simulink model "CryoDet"  (R2015b)
settings: Solver=ode45  SolverMode=SingleTasking  StartTime=0.0  StopTime=1e-4  MaxStep=1e-9  RelTol=1e-3
values from neighbouring files (symbols this model uses):
  Fclk = Fadc    (= 307200000)    [setupCryoFPGAxray.m]
  freqBusAddrBits = 4    [setupCryoFPGAxray.m]
  noise = exp(2i*pi*rand(1, noiseLen))    [setupCryoFPGAxray.m]
  noiseLen = 128    [setupCryoFPGAxray.m]
  noiseSteps = 32    [setupCryoFPGAxray.m]
  Tclk = 1/Fclk    (= 3.25520833333e-09)    [setupCryoFPGAxray.m]
undefined symbols (not defined in the file or in its folder): AXI4, Lite, notch, notch2, notch3, notch4, xlipgetpartsetting
libraries: xbsIndex_r4 x1227
(part 2 of 9)

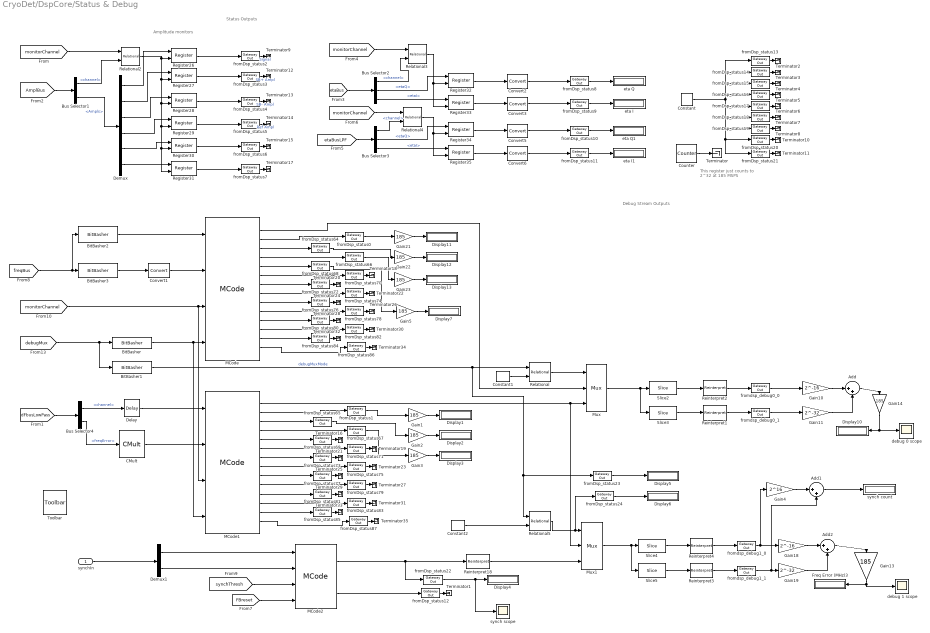
== system CryoDet/DspCore/Status & Debug ==
  note: Amplitude monitors
  note: This register just counts to 2^32 at 185 MSPS
  note: Status Outputs
  note: Debug Stream Outputs
  synchIn : Inport
  Add : Sum  Inputs=|++
  Add1 : Sum  Inputs=|++
  Add2 : Sum  Inputs=|++
  BitBasher : xbsIndex_r4/BitBasher  bitexpr=a={b[3:0]}  display_expr=on  sr_1=a  arith_type1=Unsigned  bin_pt1=0  sr_2=2  arith_type2=Unsigned  bin_pt2=0  sr_3=3  arith_type3=Unsigned  bin_pt3=0  sr_4=4  arith_type4=Unsigned  bin_pt4=0  dbl_ovrd=off  block_type=bitbasher
  BitBasher1 : xbsIndex_r4/BitBasher  bitexpr=a={b[7:4]}  display_expr=on  sr_1=a  arith_type1=Unsigned  bin_pt1=0  sr_2=2  arith_type2=Unsigned  bin_pt2=0  sr_3=3  arith_type3=Unsigned  bin_pt3=0  sr_4=4  arith_type4=Unsigned  bin_pt4=0  dbl_ovrd=off  block_type=bitbasher
  BitBasher2 : xbsIndex_r4/BitBasher  bitexpr=a={b[27:24]}  display_expr=on  sr_1=a  arith_type1=Unsigned  bin_pt1=0  sr_2=2  arith_type2=Unsigned  bin_pt2=0  sr_3=3  arith_type3=Unsigned  bin_pt3=0  sr_4=4  arith_type4=Unsigned  bin_pt4=0  dbl_ovrd=off  block_type=bitbasher
  BitBasher3 : xbsIndex_r4/BitBasher  bitexpr=a={b[23:0]}  display_expr=on  sr_1=a  arith_type1=Unsigned  bin_pt1=24  sr_2=2  arith_type2=Unsigned  bin_pt2=0  sr_3=3  arith_type3=Unsigned  bin_pt3=0  sr_4=4  arith_type4=Unsigned  bin_pt4=0  dbl_ovrd=off  block_type=bitbasher
  Bus Selector1 : BusSelector  OutputSignals=channel,Ampls
  Bus Selector2 : BusSelector  OutputSignals=channel,etaQ,etaI
  Bus Selector3 : BusSelector  OutputSignals=channel,etaQ,etaI
  Bus Selector4 : BusSelector  OutputSignals=channel,freqError
  CMult : xbsIndex_r4/CMult  const=16  gui_display_data_type=Fixed-point  const_n_bits=5  const_bin_pt=0  float_type=Single  exp_bits=8  fraction_bits=24  en=off  latency=3  precision=User Defined  arith_type="Signed  (2's comp)"  n_bits=32  bin_pt=31  quantization=Truncate  overflow=Saturate  use_behavioral_HDL=off  mem_type=Distributed RAM  pipeline=off  dbl_ovrd=off  block_type=cmult
  Constant : xbsIndex_r4/Constant  const=1.0  gui_display_data_type=Fixed-point  arith_type=Signed (2's comp)  n_bits=32  bin_pt=0  preci_type=Single  exp_width=8  frac_width=24  explicit_period=on  period=Tclk  equ=P=C  opselect=C  inp2=PCIN>>17  opr=+  inp1=P  carry=CIN  dbl_ovrd=off  block_type=constant
  Constant1 : xbsIndex_r4/Constant  const=1  gui_display_data_type=Fixed-point  arith_type=Unsigned  n_bits=4  bin_pt=0  preci_type=Single  exp_width=8  frac_width=24  explicit_period=off  period=1  equ=P=C  opselect=C  inp2=PCIN>>17  opr=+  inp1=P  carry=CIN  dbl_ovrd=off  block_type=constant
  Constant2 : xbsIndex_r4/Constant  const=0  gui_display_data_type=Fixed-point  arith_type=Unsigned  n_bits=4  bin_pt=0  preci_type=Single  exp_width=8  frac_width=24  explicit_period=off  period=1  equ=P=C  opselect=C  inp2=PCIN>>17  opr=+  inp1=P  carry=CIN  dbl_ovrd=off  block_type=constant
  Convert1 : xbsIndex_r4/Convert  gui_display_data_type=Fixed-point  arith_type="Signed  (2's comp)"  n_bits=32  bin_pt=31  float_type=Single  exp_bits=8  fraction_bits=24  quantization=Truncate  overflow=Wrap  en=off  latency=0  pipeline=off  dbl_ovrd=off  block_type=convert
  Convert{2..3,5..6} (4 alike) : xbsIndex_r4/Convert  gui_display_data_type=Fixed-point  arith_type="Signed  (2's comp)"  n_bits=32  bin_pt=14  float_type=Single  exp_bits=8  fraction_bits=24  quantization="Round  (unbiased: +/- Inf)"  overflow=Saturate  en=off  latency=1  pipeline=off  dbl_ovrd=off  block_type=convert
  Counter : xbsIndex_r4/Counter  cnt_type=Free Running  cnt_to=Inf  operation=Up  start_count=0  cnt_by_val=1  arith_type=Unsigned  n_bits=32  bin_pt=0  load_pin=off  rst=off  en=off  explicit_period=on  period=Tclk  use_behavioral_HDL=off  implementation=Fabric  dbl_ovrd=off  block_type=counter
  Delay : xbsIndex_r4/Delay  rst=off  infoeditControl=Selection of Reset will increase slice count due to use of real FFs and instead of SRLs  en=off  latency=3  reg_retiming=off  dbl_ovrd=off  block_type=delay
      settings: infoedit=Hardware notes: A delay line is a chain, each link of which is an SRL16 or SRL32 followed by a flip-flop.
  Demux : Demux  Outputs=6
  Demux1 : Demux  Outputs=2
  Display{1..7,10..13} (11 alike) : Display
      Display1 settings: Decimation=144
      Display10 settings: Decimation=144
      Display11 settings: Decimation=144
      Display12 settings: Decimation=144
      Display13 settings: Decimation=144
      Display2 settings: Decimation=144
      Display3 settings: Decimation=144
      Display7 settings: Decimation=144
  Freq Error (MHz)3 : Display
      settings: Decimation=144
  Gain{1..3,5,13..14,21..23} (9 alike) : Gain  Gain=185
  Gain10 : Gain  Gain=2^-16
  Gain11 : Gain  Gain=2^-32
  Gain18 : Gain  Gain=2^-16
  Gain19 : Gain  Gain=2^-32
  Gain4 : Gain  Gain=2^16
  MCode : xbsIndex_r4/MCode  mfname=statusAndDebugPorts  explicit_period=off  period=1  inputsTable={'boundInpExpr'=>['','','',''],'inputs'=>['Chan','f','statusMux','debugMux']}  outputsTable={'outputs'=>['debugStream','fmon','f0','f1','f2','f3','f4','f5','f6','f7','f8','f9','f10','f11'],'suppressOut'=>['off','off','off','off','off','off','off','off','off','off','off','off','off','off']}  enable_stdout=off  enable_debug=off  suppress_output=on  defparams={}  hide_port_list={}  dbl_ovrd=off  block_type=mcode
  MCode1 : xbsIndex_r4/MCode  mfname=statusAndDebugPorts  explicit_period=off  period=1  inputsTable={'boundInpExpr'=>['','','',''],'inputs'=>['Chan','f','statusMux','debugMux']}  outputsTable={'outputs'=>['debugStream','fmon','f0','f1','f2','f3','f4','f5','f6','f7','f8','f9','f10','f11'],'suppressOut'=>['off','off','off','off','off','off','off','off','off','off','off','off','off','off']}  enable_stdout=off  enable_debug=on  suppress_output=on  defparams={}  hide_port_list={}  dbl_ovrd=off  block_type=mcode
  MCode2 : xbsIndex_r4/MCode  mfname=synchronize  explicit_period=off  period=1  inputsTable={'boundInpExpr'=>['','','',''],'inputs'=>['adc0','adc1','thresh','reset']}  outputsTable={'outputs'=>['synch','minmax'],'suppressOut'=>['off','off']}  enable_stdout=off  enable_debug=off  suppress_output=on  defparams={}  hide_port_list={}  dbl_ovrd=off  block_type=mcode
  Mux : xbsIndex_r4/Mux  inputs=2  en=off  latency=0  precision=Full  arith_type=Unsigned  n_bits=16  bin_pt=14  quantization=Truncate  overflow=Wrap  dbl_ovrd=off  block_type=mux
  Mux1 : xbsIndex_r4/Mux  inputs=2  en=off  latency=0  precision=User Defined  arith_type="Signed  (2's comp)"  n_bits=32  bin_pt=31  quantization=Truncate  overflow=Saturate  dbl_ovrd=off  block_type=mux
  Register{26..35} (10 alike) : xbsIndex_r4/Register  init=0  rst=off  en=on  dbl_ovrd=off  block_type=register
  Reinterpret{1..4} (4 alike) : xbsIndex_r4/Reinterpret  force_arith_type=on  arith_type=Unsigned  force_bin_pt=off  bin_pt=15  block_type=reinterpret
  Reinterpret18 : xbsIndex_r4/Reinterpret  force_arith_type=off  arith_type=Unsigned  force_bin_pt=on  bin_pt=32  block_type=reinterpret
  Relational : xbsIndex_r4/Relational  mode=a>b  op_type=Bool  en=off  latency=0  dbl_ovrd=off  block_type=relational
  Relational2 : xbsIndex_r4/Relational  mode=a=b  op_type=Bool  en=off  latency=0  dbl_ovrd=off  block_type=relational
  Relational3 : xbsIndex_r4/Relational  mode=a=b  op_type=Bool  en=off  latency=0  dbl_ovrd=off  block_type=relational
  Relational4 : xbsIndex_r4/Relational  mode=a=b  op_type=Bool  en=off  latency=0  dbl_ovrd=off  block_type=relational
  Relational5 : xbsIndex_r4/Relational  mode=a!=b  op_type=Bool  en=off  latency=0  dbl_ovrd=off  block_type=relational
  Slice2 : xbsIndex_r4/Slice  nbits=16  boolean_output=off  mode=Upper Bit Location + Width  bit1=0  base1=MSB of Input  bit0=0  base0=LSB of Input  dbl_ovrd=off  block_type=slice
  Slice3 : xbsIndex_r4/Slice  nbits=16  boolean_output=off  mode=Lower Bit Location + Width  bit1=0  base1=MSB of Input  bit0=0  base0=LSB of Input  dbl_ovrd=off  block_type=slice
  Slice4 : xbsIndex_r4/Slice  nbits=16  boolean_output=off  mode=Upper Bit Location + Width  bit1=0  base1=MSB of Input  bit0=0  base0=LSB of Input  dbl_ovrd=off  block_type=slice
  Slice5 : xbsIndex_r4/Slice  nbits=16  boolean_output=off  mode=Lower Bit Location + Width  bit1=0  base1=MSB of Input  bit0=0  base0=LSB of Input  dbl_ovrd=off  block_type=slice
  Terminator{,1..35} (36 alike) : Terminator
  Toolbar : xbsIndex_r4/Toolbar  func=xltoolbar  block_type=toolbar
      settings: infoedit=Toolbar
  "debug 0 scope " : Scope
  debug 1 scope : Scope
  eta I : Display
      settings: Decimation=144
  eta I1 : Display
      settings: Decimation=144
  eta Q : Display
      settings: Decimation=144
  eta Q1 : Display
      settings: Decimation=144
  fromDsp_status0 : xbsIndex_r4/Gateway Out  inherit_from_input=on  hdl_port=on  rows=1  columns=1  UseAsDAC=off  DACChannel='1'  interface=AXI4-Lite  automatic_assignment=off  address_offset=hex2dec('00')  intf_name=''  intf_description=''  timing_constraint=None  locs_specified=off  LOCs={}  io_standard={}  block_type=gatewayout
  fromDsp_status1 : xbsIndex_r4/Gateway Out  inherit_from_input=on  hdl_port=on  rows=1  columns=1  UseAsDAC=off  DACChannel='1'  interface=AXI4-Lite  automatic_assignment=off  address_offset=hex2dec('04')  intf_name=''  intf_description=''  timing_constraint=None  locs_specified=off  LOCs={}  io_standard={}  block_type=gatewayout
  fromDsp_status10 : xbsIndex_r4/Gateway Out  inherit_from_input=on  hdl_port=on  rows=1  columns=1  UseAsDAC=off  DACChannel='1'  interface=AXI4-Lite  automatic_assignment=off  address_offset=hex2dec('28')  intf_name=''  intf_description=''  timing_constraint=None  locs_specified=off  LOCs={}  io_standard={}  block_type=gatewayout
  fromDsp_status11 : xbsIndex_r4/Gateway Out  inherit_from_input=on  hdl_port=on  rows=1  columns=1  UseAsDAC=off  DACChannel='1'  interface=AXI4-Lite  automatic_assignment=off  address_offset=hex2dec('2c')  intf_name=''  intf_description=''  timing_constraint=None  locs_specified=off  LOCs={}  io_standard={}  block_type=gatewayout
  fromDsp_status12 : xbsIndex_r4/Gateway Out  inherit_from_input=on  hdl_port=on  rows=1  columns=1  UseAsDAC=off  DACChannel='1'  interface=AXI4-Lite  automatic_assignment=off  address_offset=hex2dec('30')  intf_name=''  intf_description=''  timing_constraint=None  locs_specified=off  LOCs={}  io_standard={}  block_type=gatewayout
  fromDsp_status13 : xbsIndex_r4/Gateway Out  inherit_from_input=on  hdl_port=on  rows=1  columns=1  UseAsDAC=off  DACChannel='1'  interface=AXI4-Lite  automatic_assignment=off  address_offset=hex2dec('34')  intf_name=''  intf_description=''  timing_constraint=None  locs_specified=off  LOCs={}  io_standard={}  block_type=gatewayout
  fromDsp_status14 : xbsIndex_r4/Gateway Out  inherit_from_input=on  hdl_port=on  rows=1  columns=1  UseAsDAC=off  DACChannel='1'  interface=AXI4-Lite  automatic_assignment=off  address_offset=hex2dec('38')  intf_name=''  intf_description=''  timing_constraint=None  locs_specified=off  LOCs={}  io_standard={}  block_type=gatewayout
  fromDsp_status15 : xbsIndex_r4/Gateway Out  inherit_from_input=on  hdl_port=on  rows=1  columns=1  UseAsDAC=off  DACChannel='1'  interface=AXI4-Lite  automatic_assignment=off  address_offset=hex2dec('3c')  intf_name=''  intf_description=''  timing_constraint=None  locs_specified=off  LOCs={}  io_standard={}  block_type=gatewayout
  fromDsp_status16 : xbsIndex_r4/Gateway Out  inherit_from_input=on  hdl_port=on  rows=1  columns=1  UseAsDAC=off  DACChannel='1'  interface=AXI4-Lite  automatic_assignment=off  address_offset=hex2dec('40')  intf_name=''  intf_description=''  timing_constraint=None  locs_specified=off  LOCs={}  io_standard={}  block_type=gatewayout
  fromDsp_status17 : xbsIndex_r4/Gateway Out  inherit_from_input=on  hdl_port=on  rows=1  columns=1  UseAsDAC=off  DACChannel='1'  interface=AXI4-Lite  automatic_assignment=off  address_offset=hex2dec('44')  intf_name=''  intf_description=''  timing_constraint=None  locs_specified=off  LOCs={}  io_standard={}  block_type=gatewayout
  fromDsp_status18 : xbsIndex_r4/Gateway Out  inherit_from_input=on  hdl_port=on  rows=1  columns=1  UseAsDAC=off  DACChannel='1'  interface=AXI4-Lite  automatic_assignment=off  address_offset=hex2dec('48')  intf_name=''  intf_description=''  timing_constraint=None  locs_specified=off  LOCs={}  io_standard={}  block_type=gatewayout
  fromDsp_status19 : xbsIndex_r4/Gateway Out  inherit_from_input=on  hdl_port=on  rows=1  columns=1  UseAsDAC=off  DACChannel='1'  interface=AXI4-Lite  automatic_assignment=off  address_offset=hex2dec('4c')  intf_name=''  intf_description=''  timing_constraint=None  locs_specified=off  LOCs={}  io_standard={}  block_type=gatewayout
  fromDsp_status2 : xbsIndex_r4/Gateway Out  inherit_from_input=on  hdl_port=on  rows=1  columns=1  UseAsDAC=off  DACChannel='1'  interface=AXI4-Lite  automatic_assignment=off  address_offset=hex2dec('08')  intf_name=''  intf_description=''  timing_constraint=None  locs_specified=off  LOCs={}  io_standard={}  block_type=gatewayout
  fromDsp_status20 : xbsIndex_r4/Gateway Out  inherit_from_input=on  hdl_port=on  rows=1  columns=1  UseAsDAC=off  DACChannel='1'  interface=AXI4-Lite  automatic_assignment=off  address_offset=hex2dec('50')  intf_name=''  intf_description=''  timing_constraint=None  locs_specified=off  LOCs={}  io_standard={}  block_type=gatewayout
  fromDsp_status21 : xbsIndex_r4/Gateway Out  inherit_from_input=on  hdl_port=on  rows=1  columns=1  UseAsDAC=off  DACChannel='1'  interface=AXI4-Lite  automatic_assignment=off  address_offset=hex2dec('54')  intf_name=''  intf_description=''  timing_constraint=None  locs_specified=off  LOCs={}  io_standard={}  block_type=gatewayout
  fromDsp_status22 : xbsIndex_r4/Gateway Out  inherit_from_input=on  hdl_port=off  rows=1  columns=1  UseAsDAC=off  DACChannel='1'  interface=AXI4-Lite  automatic_assignment=off  address_offset=hex2dec('30')  intf_name=''  intf_description=''  timing_constraint=None  locs_specified=off  LOCs={}  io_standard={}  block_type=gatewayout
  fromDsp_status23 : xbsIndex_r4/Gateway Out  inherit_from_input=on  hdl_port=off  rows=1  columns=1  UseAsDAC=off  DACChannel='1'  interface=AXI4-Lite  automatic_assignment=off  address_offset=hex2dec('30')  intf_name=''  intf_description=''  timing_constraint=None  locs_specified=off  LOCs={}  io_standard={}  block_type=gatewayout
  fromDsp_status24 : xbsIndex_r4/Gateway Out  inherit_from_input=on  hdl_port=off  rows=1  columns=1  UseAsDAC=off  DACChannel='1'  interface=AXI4-Lite  automatic_assignment=off  address_offset=hex2dec('30')  intf_name=''  intf_description=''  timing_constraint=None  locs_specified=off  LOCs={}  io_standard={}  block_type=gatewayout
  fromDsp_status3 : xbsIndex_r4/Gateway Out  inherit_from_input=on  hdl_port=on  rows=1  columns=1  UseAsDAC=off  DACChannel='1'  interface=AXI4-Lite  automatic_assignment=off  address_offset=hex2dec('0C')  intf_name=''  intf_description=''  timing_constraint=None  locs_specified=off  LOCs={}  io_standard={}  block_type=gatewayout
  fromDsp_status4 : xbsIndex_r4/Gateway Out  inherit_from_input=on  hdl_port=on  rows=1  columns=1  UseAsDAC=off  DACChannel='1'  interface=AXI4-Lite  automatic_assignment=off  address_offset=hex2dec('10')  intf_name=''  intf_description=''  timing_constraint=None  locs_specified=off  LOCs={}  io_standard={}  block_type=gatewayout
  fromDsp_status5 : xbsIndex_r4/Gateway Out  inherit_from_input=on  hdl_port=on  rows=1  columns=1  UseAsDAC=off  DACChannel='1'  interface=AXI4-Lite  automatic_assignment=off  address_offset=hex2dec('14')  intf_name=''  intf_description=''  timing_constraint=None  locs_specified=off  LOCs={}  io_standard={}  block_type=gatewayout
  fromDsp_status6 : xbsIndex_r4/Gateway Out  inherit_from_input=on  hdl_port=on  rows=1  columns=1  UseAsDAC=off  DACChannel='1'  interface=AXI4-Lite  automatic_assignment=off  address_offset=hex2dec('18')  intf_name=''  intf_description=''  timing_constraint=None  locs_specified=off  LOCs={}  io_standard={}  block_type=gatewayout
  fromDsp_status64 : xbsIndex_r4/Gateway Out  inherit_from_input=on  hdl_port=on  rows=1  columns=1  UseAsDAC=off  DACChannel='1'  interface=AXI4-Lite  automatic_assignment=off  address_offset=hex2dec('100')  intf_name=''  intf_description=''  timing_constraint=None  locs_specified=off  LOCs={}  io_standard={}  block_type=gatewayout
  fromDsp_status65 : xbsIndex_r4/Gateway Out  inherit_from_input=on  hdl_port=on  rows=1  columns=1  UseAsDAC=off  DACChannel='1'  interface=AXI4-Lite  automatic_assignment=off  address_offset=hex2dec('104')  intf_name=''  intf_description=''  timing_constraint=None  locs_specified=off  LOCs={}  io_standard={}  block_type=gatewayout
  fromDsp_status66 : xbsIndex_r4/Gateway Out  inherit_from_input=on  hdl_port=on  rows=1  columns=1  UseAsDAC=off  DACChannel='1'  interface=AXI4-Lite  automatic_assignment=off  address_offset=hex2dec('108')  intf_name=''  intf_description=''  timing_constraint=None  locs_specified=off  LOCs={}  io_standard={}  block_type=gatewayout
  fromDsp_status67 : xbsIndex_r4/Gateway Out  inherit_from_input=on  hdl_port=on  rows=1  columns=1  UseAsDAC=off  DACChannel='1'  interface=AXI4-Lite  automatic_assignment=off  address_offset=hex2dec('10c')  intf_name=''  intf_description=''  timing_constraint=None  locs_specified=off  LOCs={}  io_standard={}  block_type=gatewayout
  fromDsp_status68 : xbsIndex_r4/Gateway Out  inherit_from_input=on  hdl_port=on  rows=1  columns=1  UseAsDAC=off  DACChannel='1'  interface=AXI4-Lite  automatic_assignment=off  address_offset=hex2dec('110')  intf_name=''  intf_description=''  timing_constraint=None  locs_specified=off  LOCs={}  io_standard={}  block_type=gatewayout
  fromDsp_status69 : xbsIndex_r4/Gateway Out  inherit_from_input=on  hdl_port=on  rows=1  columns=1  UseAsDAC=off  DACChannel='1'  interface=AXI4-Lite  automatic_assignment=off  address_offset=hex2dec('114')  intf_name=''  intf_description=''  timing_constraint=None  locs_specified=off  LOCs={}  io_standard={}  block_type=gatewayout
  fromDsp_status7 : xbsIndex_r4/Gateway Out  inherit_from_input=on  hdl_port=on  rows=1  columns=1  UseAsDAC=off  DACChannel='1'  interface=AXI4-Lite  automatic_assignment=off  address_offset=hex2dec('1C')  intf_name=''  intf_description=''  timing_constraint=None  locs_specified=off  LOCs={}  io_standard={}  block_type=gatewayout
  fromDsp_status70 : xbsIndex_r4/Gateway Out  inherit_from_input=on  hdl_port=on  rows=1  columns=1  UseAsDAC=off  DACChannel='1'  interface=AXI4-Lite  automatic_assignment=off  address_offset=hex2dec('118')  intf_name=''  intf_description=''  timing_constraint=None  locs_specified=off  LOCs={}  io_standard={}  block_type=gatewayout
  fromDsp_status71 : xbsIndex_r4/Gateway Out  inherit_from_input=on  hdl_port=on  rows=1  columns=1  UseAsDAC=off  DACChannel='1'  interface=AXI4-Lite  automatic_assignment=off  address_offset=hex2dec('11c')  intf_name=''  intf_description=''  timing_constraint=None  locs_specified=off  LOCs={}  io_standard={}  block_type=gatewayout
  fromDsp_status72 : xbsIndex_r4/Gateway Out  inherit_from_input=on  hdl_port=on  rows=1  columns=1  UseAsDAC=off  DACChannel='1'  interface=AXI4-Lite  automatic_assignment=off  address_offset=hex2dec('120')  intf_name=''  intf_description=''  timing_constraint=None  locs_specified=off  LOCs={}  io_standard={}  block_type=gatewayout
  fromDsp_status73 : xbsIndex_r4/Gateway Out  inherit_from_input=on  hdl_port=on  rows=1  columns=1  UseAsDAC=off  DACChannel='1'  interface=AXI4-Lite  automatic_assignment=off  address_offset=hex2dec('124')  intf_name=''  intf_description=''  timing_constraint=None  locs_specified=off  LOCs={}  io_standard={}  block_type=gatewayout
  fromDsp_status74 : xbsIndex_r4/Gateway Out  inherit_from_input=on  hdl_port=on  rows=1  columns=1  UseAsDAC=off  DACChannel='1'  interface=AXI4-Lite  automatic_assignment=off  address_offset=hex2dec('128')  intf_name=''  intf_description=''  timing_constraint=None  locs_specified=off  LOCs={}  io_standard={}  block_type=gatewayout
  fromDsp_status75 : xbsIndex_r4/Gateway Out  inherit_from_input=on  hdl_port=on  rows=1  columns=1  UseAsDAC=off  DACChannel='1'  interface=AXI4-Lite  automatic_assignment=off  address_offset=hex2dec('12c')  intf_name=''  intf_description=''  timing_constraint=None  locs_specified=off  LOCs={}  io_standard={}  block_type=gatewayout
  fromDsp_status76 : xbsIndex_r4/Gateway Out  inherit_from_input=on  hdl_port=on  rows=1  columns=1  UseAsDAC=off  DACChannel='1'  interface=AXI4-Lite  automatic_assignment=off  address_offset=hex2dec('130')  intf_name=''  intf_description=''  timing_constraint=None  locs_specified=off  LOCs={}  io_standard={}  block_type=gatewayout
  fromDsp_status77 : xbsIndex_r4/Gateway Out  inherit_from_input=on  hdl_port=on  rows=1  columns=1  UseAsDAC=off  DACChannel='1'  interface=AXI4-Lite  automatic_assignment=off  address_offset=hex2dec('134')  intf_name=''  intf_description=''  timing_constraint=None  locs_specified=off  LOCs={}  io_standard={}  block_type=gatewayout
  fromDsp_status78 : xbsIndex_r4/Gateway Out  inherit_from_input=on  hdl_port=on  rows=1  columns=1  UseAsDAC=off  DACChannel='1'  interface=AXI4-Lite  automatic_assignment=off  address_offset=hex2dec('138')  intf_name=''  intf_description=''  timing_constraint=None  locs_specified=off  LOCs={}  io_standard={}  block_type=gatewayout
  fromDsp_status79 : xbsIndex_r4/Gateway Out  inherit_from_input=on  hdl_port=on  rows=1  columns=1  UseAsDAC=off  DACChannel='1'  interface=AXI4-Lite  automatic_assignment=off  address_offset=hex2dec('13c')  intf_name=''  intf_description=''  timing_constraint=None  locs_specified=off  LOCs={}  io_standard={}  block_type=gatewayout
  fromDsp_status8 : xbsIndex_r4/Gateway Out  inherit_from_input=on  hdl_port=on  rows=1  columns=1  UseAsDAC=off  DACChannel='1'  interface=AXI4-Lite  automatic_assignment=off  address_offset=hex2dec('20')  intf_name=''  intf_description=''  timing_constraint=None  locs_specified=off  LOCs={}  io_standard={}  block_type=gatewayout
  fromDsp_status80 : xbsIndex_r4/Gateway Out  inherit_from_input=on  hdl_port=on  rows=1  columns=1  UseAsDAC=off  DACChannel='1'  interface=AXI4-Lite  automatic_assignment=off  address_offset=hex2dec('140')  intf_name=''  intf_description=''  timing_constraint=None  locs_specified=off  LOCs={}  io_standard={}  block_type=gatewayout
  fromDsp_status81 : xbsIndex_r4/Gateway Out  inherit_from_input=on  hdl_port=on  rows=1  columns=1  UseAsDAC=off  DACChannel='1'  interface=AXI4-Lite  automatic_assignment=off  address_offset=hex2dec('144')  intf_name=''  intf_description=''  timing_constraint=None  locs_specified=off  LOCs={}  io_standard={}  block_type=gatewayout
  fromDsp_status82 : xbsIndex_r4/Gateway Out  inherit_from_input=on  hdl_port=on  rows=1  columns=1  UseAsDAC=off  DACChannel='1'  interface=AXI4-Lite  automatic_assignment=off  address_offset=hex2dec('148')  intf_name=''  intf_description=''  timing_constraint=None  locs_specified=off  LOCs={}  io_standard={}  block_type=gatewayout
  fromDsp_status83 : xbsIndex_r4/Gateway Out  inherit_from_input=on  hdl_port=on  rows=1  columns=1  UseAsDAC=off  DACChannel='1'  interface=AXI4-Lite  automatic_assignment=off  address_offset=hex2dec('14c')  intf_name=''  intf_description=''  timing_constraint=None  locs_specified=off  LOCs={}  io_standard={}  block_type=gatewayout
  fromDsp_status84 : xbsIndex_r4/Gateway Out  inherit_from_input=on  hdl_port=on  rows=1  columns=1  UseAsDAC=off  DACChannel='1'  interface=AXI4-Lite  automatic_assignment=off  address_offset=hex2dec('150')  intf_name=''  intf_description=''  timing_constraint=None  locs_specified=off  LOCs={}  io_standard={}  block_type=gatewayout
  fromDsp_status85 : xbsIndex_r4/Gateway Out  inherit_from_input=on  hdl_port=on  rows=1  columns=1  UseAsDAC=off  DACChannel='1'  interface=AXI4-Lite  automatic_assignment=off  address_offset=hex2dec('154')  intf_name=''  intf_description=''  timing_constraint=None  locs_specified=off  LOCs={}  io_standard={}  block_type=gatewayout
  fromDsp_status86 : xbsIndex_r4/Gateway Out  inherit_from_input=on  hdl_port=on  rows=1  columns=1  UseAsDAC=off  DACChannel='1'  interface=AXI4-Lite  automatic_assignment=off  address_offset=hex2dec('158')  intf_name=''  intf_description=''  timing_constraint=None  locs_specified=off  LOCs={}  io_standard={}  block_type=gatewayout
  fromDsp_status87 : xbsIndex_r4/Gateway Out  inherit_from_input=on  hdl_port=on  rows=1  columns=1  UseAsDAC=off  DACChannel='1'  interface=AXI4-Lite  automatic_assignment=off  address_offset=hex2dec('15c')  intf_name=''  intf_description=''  timing_constraint=None  locs_specified=off  LOCs={}  io_standard={}  block_type=gatewayout
  fromDsp_status9 : xbsIndex_r4/Gateway Out  inherit_from_input=on  hdl_port=on  rows=1  columns=1  UseAsDAC=off  DACChannel='1'  interface=AXI4-Lite  automatic_assignment=off  address_offset=hex2dec('24')  intf_name=''  intf_description=''  timing_constraint=None  locs_specified=off  LOCs={}  io_standard={}  block_type=gatewayout
  fromdsp_debug0_0 : xbsIndex_r4/Gateway Out  inherit_from_input=on  hdl_port=on  rows=1  columns=1  UseAsDAC=off  DACChannel='1'  interface=None  automatic_assignment=on  address_offset=hex2dec('00')  intf_name=''  intf_description=''  timing_constraint=None  locs_specified=off  LOCs={}  io_standard={}  block_type=gatewayout
  fromdsp_debug0_1 : xbsIndex_r4/Gateway Out  inherit_from_input=on  hdl_port=on  rows=1  columns=1  UseAsDAC=off  DACChannel='1'  interface=None  automatic_assignment=on  address_offset=hex2dec('00')  intf_name=''  intf_description=''  timing_constraint=None  locs_specified=off  LOCs={}  io_standard={}  block_type=gatewayout
  fromdsp_debug1_0 : xbsIndex_r4/Gateway Out  inherit_from_input=on  hdl_port=on  rows=1  columns=1  UseAsDAC=off  DACChannel='1'  interface=None  automatic_assignment=on  address_offset=hex2dec('00')  intf_name=''  intf_description=''  timing_constraint=None  locs_specified=off  LOCs={}  io_standard={}  block_type=gatewayout
  fromdsp_debug1_1 : xbsIndex_r4/Gateway Out  inherit_from_input=off  hdl_port=on  rows=1  columns=1  UseAsDAC=off  DACChannel='1'  interface=None  automatic_assignment=on  address_offset=hex2dec('00')  intf_name=''  intf_description=''  timing_constraint=None  locs_specified=off  LOCs={}  io_standard={}  block_type=gatewayout
  synch count : Display
  synch scope : Scope
  wires:
  Register28/1 -> fromDsp_status4/1
  Register27/1 -> fromDsp_status3/1
  Register26/1 -> fromDsp_status2/1
  fromdsp_debug0_1/1 -> Gain11/1
  fromdsp_debug0_0/1 -> Gain10/1
  [monitorChannel] -> Relational2/1
  Slice3/1 -> Reinterpret1/1
  Reinterpret2/1 -> fromdsp_debug0_0/1
  Slice2/1 -> Reinterpret2/1
  Reinterpret1/1 -> fromdsp_debug0_1/1
  Gain14/1 -> Display10/1, "debug 0 scope "/1
  Gain10/1 -> Add/1
  Add/1 -> Gain14/1
  Gain11/1 -> Add/2
  Register29/1 -> fromDsp_status5/1
  Register30/1 -> fromDsp_status6/1
  Register31/1 -> fromDsp_status7/1
  [AmplBus] -> Bus Selector1/1
  Bus Selector1/1 -> Relational2/2  "<channel>"
  Relational2/1 -> Register27/2, Register28/2, Register29/2, Register30/2, Register31/2, Register26/2
  Demux/6 -> Register31/1
  Demux/5 -> Register30/1
  Demux/4 -> Register29/1
  Demux/3 -> Register28/1
  Demux/2 -> Register27/1
  Demux/1 -> Register26/1
  Bus Selector1/2 -> Demux/1  "<Ampls>"
  [etaBus] -> Bus Selector2/1
  Register32/1 -> Convert2/1
  Register33/1 -> Convert3/1
  [monitorChannel] -> Relational3/1
  Bus Selector2/1 -> Relational3/2  "<channel>"
  Bus Selector2/2 -> Register32/1  "<etaQ>"
  Bus Selector2/3 -> Register33/1  "<etaI>"
  Relational3/1 -> Register33/2, Register32/2
  fromDsp_status8/1 -> eta Q/1
  fromDsp_status9/1 -> eta I/1
  Convert2/1 -> fromDsp_status8/1
  Convert3/1 -> fromDsp_status9/1
  Register34/1 -> Convert5/1
  Register35/1 -> Convert6/1
  Bus Selector3/1 -> Relational4/2  "<channel>"
  Bus Selector3/2 -> Register34/1  "<etaQ>"
  Bus Selector3/3 -> Register35/1  "<etaI>"
  Relational4/1 -> Register35/2, Register34/2
  fromDsp_status10/1 -> eta Q1/1
  fromDsp_status11/1 -> eta I1/1
  Convert5/1 -> fromDsp_status10/1
  Convert6/1 -> fromDsp_status11/1
  [etaBusLPF] -> Bus Selector3/1
  [monitorChannel] -> Relational4/1
  Constant/1 -> fromDsp_status13/1, fromDsp_status14/1, fromDsp_status15/1, fromDsp_status16/1, fromDsp_status17/1, fromDsp_status18/1, fromDsp_status19/1, fromDsp_status21/1, fromDsp_status20/1
  Slice5/1 -> Reinterpret3/1
  Reinterpret4/1 -> fromdsp_debug1_0/1
  Slice4/1 -> Reinterpret4/1
  Reinterpret3/1 -> fromdsp_debug1_1/1
  Gain18/1 -> Add2/1
  Gain19/1 -> Add2/2
  Add2/1 -> Gain13/1
  Gain13/1 -> debug 1 scope/1, Freq Error (MHz)3/1
  [freqBus] -> BitBasher2/1, BitBasher3/1
  BitBasher2/1 -> MCode/1
  BitBasher3/1 -> Convert1/1
  Convert1/1 -> MCode/2
  [monitorChannel] -> MCode1/3, MCode/3
  [debugMux] -> BitBasher1/1, BitBasher/1
  [dFbusLowPass] -> Bus Selector4/1
  Bus Selector4/1 -> Delay/1  "<channel>"
  Bus Selector4/2 -> CMult/1  "<freqError>"
  MCode/13 -> fromDsp_status84/1
  MCode/11 -> fromDsp_status80/1
  MCode/9 -> fromDsp_status76/1
  MCode/7 -> fromDsp_status72/1
  MCode/5 -> fromDsp_status68/1
  MCode/3 -> fromDsp_status64/1
  MCode/12 -> fromDsp_status82/1
  MCode/10 -> fromDsp_status78/1
  MCode/8 -> fromDsp_status74/1
  MCode/6 -> fromDsp_status70/1
  MCode/4 -> fromDsp_status66/1
  MCode/2 -> fromDsp_status0/1
  MCode/14 -> fromDsp_status86/1
  Gain21/1 -> Display11/1
  Gain22/1 -> Display12/1
  Gain23/1 -> Display13/1
  fromDsp_status0/1 -> Gain21/1
  fromDsp_status64/1 -> Gain22/1
  fromDsp_status66/1 -> Gain23/1
  CMult/1 -> MCode1/2
  Counter/1 -> Terminator/1
  Demux1/1 -> MCode2/1
  Demux1/2 -> MCode2/2
  synchIn/1 -> Demux1/1
  BitBasher/1 -> MCode1/4, MCode/4
  MCode/1 -> Mux/2
  MCode1/1 -> Mux/3, Mux1/2
  BitBasher1/1 -> Relational5/1, fromDsp_status23/1, Relational/1  "debugMuxMode"
  Relational/1 -> Mux/1
  Constant1/1 -> Relational/2
  Constant2/1 -> Relational5/2
  Relational5/1 -> fromDsp_status24/1, Mux1/1
  Mux/1 -> Slice3/1, Slice2/1
  Mux1/1 -> Slice5/1, Slice4/1
  [FBreset] -> MCode2/4
  [synchThresh] -> MCode2/3
  MCode2/2 -> fromDsp_status12/1
  Gain1/1 -> Display1/1
  Gain2/1 -> Display2/1
  Gain3/1 -> Display3/1
  fromDsp_status1/1 -> Gain1/1
  fromDsp_status65/1 -> Gain2/1
  fromDsp_status67/1 -> Gain3/1
  MCode1/2 -> fromDsp_status1/1
  MCode1/3 -> fromDsp_status65/1
  MCode1/4 -> fromDsp_status67/1
  MCode1/5 -> fromDsp_status69/1
  MCode1/6 -> fromDsp_status71/1
  MCode1/7 -> fromDsp_status73/1
  MCode1/14 -> fromDsp_status87/1
  MCode1/13 -> fromDsp_status85/1
  MCode1/12 -> fromDsp_status83/1
  MCode1/11 -> fromDsp_status81/1
  MCode1/10 -> fromDsp_status79/1
  MCode1/9 -> fromDsp_status77/1
  MCode1/8 -> fromDsp_status75/1
  MCode2/1 -> fromDsp_status22/1, Reinterpret18/1
  fromDsp_status22/1 -> synch scope/1, Display4/1
  fromDsp_status23/1 -> Display5/1
  fromDsp_status24/1 -> Display6/1
  Reinterpret18/1 -> Mux1/3
  fromdsp_debug1_0/1 -> Gain4/1, Gain18/1
  Gain4/1 -> Add1/1
  fromdsp_debug1_1/1 -> Add1/2, Gain19/1
  Add1/1 -> synch count/1
  Gain5/1 -> Display7/1
  fromDsp_status68/1 -> Gain5/1
  fromDsp_status12/1 -> Terminator1/1
  fromDsp_status13/1 -> Terminator2/1
  fromDsp_status14/1 -> Terminator3/1
  fromDsp_status15/1 -> Terminator4/1
  fromDsp_status16/1 -> Terminator5/1
  fromDsp_status17/1 -> Terminator6/1
  fromDsp_status18/1 -> Terminator7/1
  fromDsp_status19/1 -> Terminator8/1
  fromDsp_status2/1 -> Terminator9/1  "Signal"
  fromDsp_status20/1 -> Terminator10/1
  fromDsp_status21/1 -> Terminator11/1
  fromDsp_status3/1 -> Terminator12/1  "SB+ Ampl"
  fromDsp_status4/1 -> Terminator13/1  "SB- Ampl"
  fromDsp_status5/1 -> Terminator14/1  "Ref Ampl"
  fromDsp_status6/1 -> Terminator15/1
  fromDsp_status69/1 -> Terminator16/1
  fromDsp_status7/1 -> Terminator17/1
  fromDsp_status70/1 -> Terminator18/1
  fromDsp_status71/1 -> Terminator19/1
  fromDsp_status72/1 -> Terminator20/1
  fromDsp_status73/1 -> Terminator21/1
  fromDsp_status74/1 -> Terminator22/1
  fromDsp_status75/1 -> Terminator23/1
  fromDsp_status76/1 -> Terminator24/1
  fromDsp_status77/1 -> Terminator25/1
  fromDsp_status78/1 -> Terminator26/1
  fromDsp_status79/1 -> Terminator27/1
  fromDsp_status80/1 -> Terminator28/1
  fromDsp_status81/1 -> Terminator29/1
  fromDsp_status82/1 -> Terminator30/1
  fromDsp_status83/1 -> Terminator31/1
  fromDsp_status84/1 -> Terminator32/1
  fromDsp_status85/1 -> Terminator33/1
  fromDsp_status86/1 -> Terminator34/1
  fromDsp_status87/1 -> Terminator35/1
  Delay/1 -> MCode1/1

== system CryoDet/DspCore/AdcDac 0/Amplitudes ==
  note: tvalid
  note: Channel #
  note: Sig+
  note: Sig-
  note: Ref+
  note: Ref
  note: Sig
  note: Ref-
  In2 : Inport
  Ampl Scope : Scope  NumInputPorts=5
  Bus Creator : BusCreator  Inputs=3
  Bus Selector1 : BusSelector  OutputSignals=channel&tvalid,I&Qlpf
  Bus Selector2 : BusSelector  OutputSignals=channel,tvalid
  CORDIC 6.0 {,1..5} (6 alike) : xbsIndex_r4/CORDIC 6.0   functional_selection=Translate  architectural_configuration=Parallel  pipelining_mode=Optimal  data_format=SignedFraction  phase_format=Scaled_Radians  input_width=24  output_width=20  round_mode=Truncate  iterations=0  precision=0  compensation_scaling=Embedded_Multiplier  coarse_rotation=on  aclken=off  aresetn=off  out_tready=off  cartesian_has_tuser=off  cartesian_has_tlast=off  cartesian_tuser_width=1  phase_has_tuser=off  phase_has_tlast=off  phase_tuser_width=1  out_tlast_behv=Null  flow_control=Blocking  optimize_goal=Resources  trim_axipin_name=on  simulation_type=hybrid_sim  simulation_model=sysgen:cordic_v6_0  data_path_portlist={'s_axis_cartesian_tdata_imag', 's_axis_cartesian_tdata_real', 's_axis_phase_tdata_phase', 'm_axis_dout_tdata_imag', 'm_axis_dout_tdata_real', 'm_axis_dout_tdata_phase','m_axis_dout_tdata'}  ip_name=CORDIC  ip_version=6.0  dsptool_ready=true  ipcore_usecache=true  ipcore_useipmodelcache=true  wrapper_available=true  port_translation_map={ 'aclken' => 'en', 'aresetn' => 'rst' }  block_type=cordic_v6_0
      settings: infoedit=CORDIC 6.0
  Constant : xbsIndex_r4/Constant  const=1  gui_display_data_type=Boolean  arith_type=Boolean  n_bits=16  bin_pt=14  preci_type=Single  exp_width=8  frac_width=24  explicit_period=off  period=1  equ=P=C  opselect=C  inp2=PCIN>>17  opr=+  inp1=P  carry=CIN  dbl_ovrd=off  block_type=constant
  Delay : xbsIndex_r4/Delay  rst=off  infoeditControl=Selection of Reset will increase slice count due to use of real FFs and instead of SRLs  en=off  latency=28  reg_retiming=off  dbl_ovrd=off  block_type=delay
  Delay1 : xbsIndex_r4/Delay  rst=off  infoeditControl=Selection of Reset will increase slice count due to use of real FFs and instead of SRLs  en=off  latency=28  reg_retiming=off  dbl_ovrd=off  block_type=delay
  Demux{1,13,15..18} (6 alike) : Demux  Outputs=2
  Demux14 : Demux  Outputs=6
  Gateway Out{,1..7} (8 alike) : xbsIndex_r4/Gateway Out  inherit_from_input=off  hdl_port=off  rows=1  columns=1  UseAsDAC=off  DACChannel='1'  interface=None  automatic_assignment=on  address_offset=hex2dec('00')  intf_name=''  intf_description=''  timing_constraint=None  locs_specified=off  LOCs={}  io_standard={}  block_type=gatewayout
  Mux : Mux  Inputs=6
  Mux1 : Mux  Inputs=2
  Mux2 : Mux  Inputs=2
  Mux3 : Mux  Inputs=2
  Terminator{,1..17} (18 alike) : Terminator
  tag scope: AmplBus=global
  wires:
  Demux14/2 -> Demux13/1
  Demux14/3 -> Demux15/1
  Demux14/5 -> Demux17/1
  Demux14/6 -> Demux18/1
  Bus Selector1/2 -> Demux14/1  "<I&Qlpf>"
  In2/1 -> Bus Selector1/1
  Demux14/4 -> Demux16/1
  Bus Selector2/1 -> Delay/1  "<channel>"
  Bus Selector1/1 -> Bus Selector2/1  "<channel&tvalid>"
  Demux14/1 -> Demux1/1
  Demux1/2 -> "CORDIC 6.0 "/3
  Demux1/1 -> "CORDIC 6.0 "/2
  Demux18/1 -> CORDIC 6.0 5/2
  Demux18/2 -> CORDIC 6.0 5/3
  Demux17/1 -> CORDIC 6.0 4/2
  Demux17/2 -> CORDIC 6.0 4/3
  Demux16/1 -> CORDIC 6.0 3/2
  Demux16/2 -> CORDIC 6.0 3/3
  Demux15/1 -> CORDIC 6.0 2/2
  Demux15/2 -> CORDIC 6.0 2/3
  Demux13/1 -> CORDIC 6.0 1/2
  Demux13/2 -> CORDIC 6.0 1/3
  Constant/1 -> CORDIC 6.0 1/1, CORDIC 6.0 2/1, CORDIC 6.0 3/1, CORDIC 6.0 4/1, CORDIC 6.0 5/1, "CORDIC 6.0 "/1
  Bus Selector2/2 -> Delay1/1  "<tvalid>"
  Delay/1 -> Gateway Out/1, Bus Creator/1  "channel"
  Delay1/1 -> Gateway Out1/1, Bus Creator/2  "tvalid"
  "CORDIC 6.0 "/4 -> Gateway Out2/1, Mux/1
  CORDIC 6.0 1/4 -> Mux/2, Gateway Out3/1
  CORDIC 6.0 2/4 -> Gateway Out4/1, Mux/3
  CORDIC 6.0 3/4 -> Gateway Out5/1, Mux/4
  CORDIC 6.0 4/4 -> Gateway Out6/1, Mux/5
  CORDIC 6.0 5/4 -> Gateway Out7/1, Mux/6
  Bus Creator/1 -> [AmplBus]
  Mux/1 -> Bus Creator/3  "Ampls"
  Gateway Out/1 -> Mux1/1
  Gateway Out1/1 -> Mux1/2
  Gateway Out3/1 -> Mux2/1
  Gateway Out4/1 -> Mux2/2
  Mux1/1 -> Ampl Scope/1
  Gateway Out2/1 -> Ampl Scope/2
  Mux2/1 -> Ampl Scope/3
  Gateway Out5/1 -> Ampl Scope/4
  Gateway Out6/1 -> Mux3/1
  Gateway Out7/1 -> Mux3/2
  Mux3/1 -> Ampl Scope/5
  "CORDIC 6.0 "/1 -> Terminator/1
  "CORDIC 6.0 "/2 -> Terminator1/1
  "CORDIC 6.0 "/3 -> Terminator2/1
  CORDIC 6.0 1/1 -> Terminator3/1
  CORDIC 6.0 1/2 -> Terminator4/1
  CORDIC 6.0 1/3 -> Terminator5/1
  CORDIC 6.0 2/1 -> Terminator6/1
  CORDIC 6.0 2/2 -> Terminator7/1
  CORDIC 6.0 2/3 -> Terminator8/1
  CORDIC 6.0 3/1 -> Terminator9/1
  CORDIC 6.0 3/2 -> Terminator10/1
  CORDIC 6.0 3/3 -> Terminator11/1
  CORDIC 6.0 4/1 -> Terminator12/1
  CORDIC 6.0 4/2 -> Terminator13/1
  CORDIC 6.0 4/3 -> Terminator14/1
  CORDIC 6.0 5/1 -> Terminator15/1
  CORDIC 6.0 5/2 -> Terminator16/1
  CORDIC 6.0 5/3 -> Terminator17/1

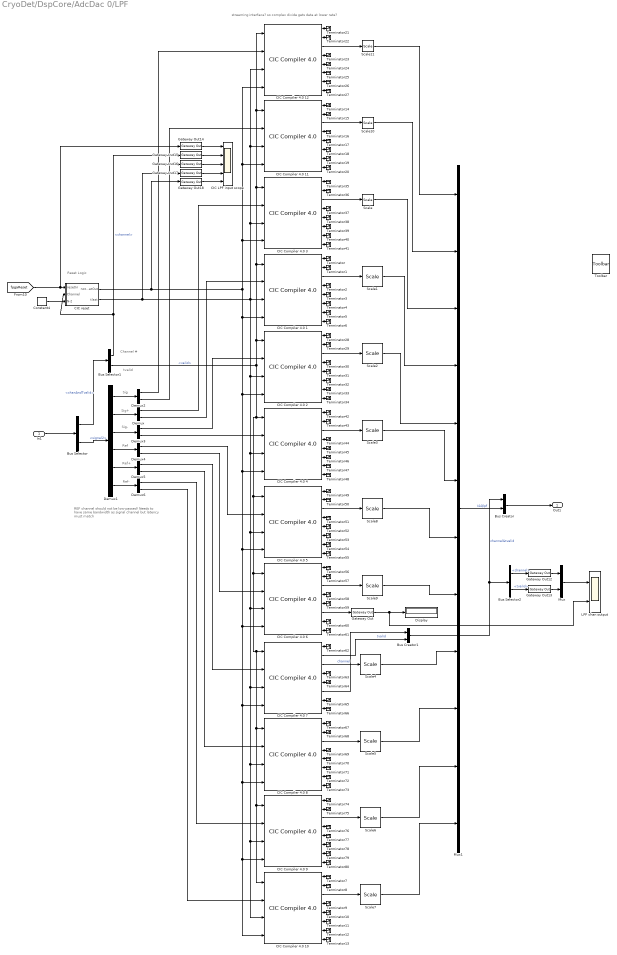
== system CryoDet/DspCore/AdcDac 0/LPF ==
  note: Reset Logic
  note: REF channel should not be low-passed!
      | Needs to have same bandwidth as signal channel
      | but latency must match
  note: streaming interface? so complex divide gets data at lower rate?
  note: tvalid
  note: Channel #
  note: Sig+
  note: Sig-
  note: Ref+
  note: Ref
  note: Sig
  note: Ref-
  In1 : Inport
  Bus Creator : BusCreator  Inputs=2
  Bus Creator1 : BusCreator  Inputs=2
  Bus Selector : BusSelector  OutputSignals=chanAndTvalid,signal2
  Bus Selector1 : BusSelector  OutputSignals=channel,valid
  Bus Selector2 : BusSelector  OutputSignals=channel,tvalid
  CIC Compiler 4.0 {1..12} (12 alike) : xbsIndex_r4/CIC Compiler 4.0   filter_type=Decimation  number_of_stages=3  differential_delay=1  number_of_channels=12  sample_rate_changes=Fixed  fixed_or_initial_rate=8  minimum_rate=8  maximum_rate=8  ratespecification=Sample_Period  sampleperiod=1  hardwareoversamplingrate=1  quantization=Truncation  output_data_width=24  use_xtreme_dsp_slice=off  use_streaming_interface=on  has_aclken=off  has_aresetn=on  has_dout_tready=off  trim_axipin_name=on  gui_behaviour=Sysgen_GUI  input_data_width=18  ip_name=CIC Compiler  ip_version=4.0  dsptool_ready=true  wrapper_available=true  port_translation_map={ 'aclken' => 'en', 'aresetn' => 'rst' }  ipcore_xco_need_fpga_part=true  ipcore_verbose=false  block_type=cic_compiler_v4_0
  CIC LPF input scope : Scope  NumInputPorts=5
  CIC reset : Subsystem
  Constant4 : xbsIndex_r4/Constant  const=10  gui_display_data_type=Fixed-point  arith_type=Unsigned  n_bits=4  bin_pt=0  preci_type=Single  exp_width=8  frac_width=24  explicit_period=off  period=1  equ=P=C  opselect=C  inp2=PCIN>>17  opr=+  inp1=P  carry=CIN  dbl_ovrd=off  block_type=constant
  Demux{,2..6} (6 alike) : Demux  Outputs=2
  Demux1 : Demux  Outputs=6
  Display : Display
  Gateway Out{,12..18} (8 alike) : xbsIndex_r4/Gateway Out  inherit_from_input=off  hdl_port=off  rows=1  columns=1  UseAsDAC=off  DACChannel='1'  interface=None  automatic_assignment=on  address_offset=hex2dec('00')  intf_name=''  intf_description=''  timing_constraint=None  locs_specified=off  LOCs={}  io_standard={}  block_type=gatewayout
  LPF chan output : Scope  NumInputPorts=2
  Mux : Mux  Inputs=2
  Mux1 : Mux  Inputs=12
  Scale{,1..11} (12 alike) : xbsIndex_r4/Scale  scale_factor=-9  dbl_ovrd=off  block_type=scale
  Terminator{,1..80} (81 alike) : Terminator
  Toolbar : xbsIndex_r4/Toolbar  func=xltoolbar  block_type=toolbar
      settings: infoedit=Toolbar
  Out1 : Outport
  wires:
  Demux1/1 -> Demux2/1
  Demux1/2 -> Demux/1
  Demux1/3 -> Demux3/1
  Demux1/5 -> Demux5/1
  Demux1/6 -> Demux6/1
  Bus Selector/2 -> Demux1/1  "<signal2>"
  In1/1 -> Bus Selector/1
  Demux1/4 -> Demux4/1
  Demux/1 -> CIC Compiler 4.0 3/2
  Demux/2 -> CIC Compiler 4.0 1/2
  Demux3/1 -> CIC Compiler 4.0 2/2
  Demux3/2 -> CIC Compiler 4.0 4/2
  Demux5/1 -> CIC Compiler 4.0 7/2
  Demux5/2 -> CIC Compiler 4.0 8/2
  Demux6/1 -> CIC Compiler 4.0 9/2
  Demux6/2 -> CIC Compiler 4.0 10/2
  Bus Selector1/2 -> CIC Compiler 4.0 11/1, CIC Compiler 4.0 12/1, CIC Compiler 4.0 3/1, CIC Compiler 4.0 1/1, CIC Compiler 4.0 2/1, CIC Compiler 4.0 4/1, CIC Compiler 4.0 5/1, CIC Compiler 4.0 6/1, CIC Compiler 4.0 7/1, CIC Compiler 4.0 8/1, CIC Compiler 4.0 9/1, CIC Compiler 4.0 10/1  "<valid>"
  Bus Selector1/1 -> Gateway Out15/1, CIC reset/2(Channel)  "<channel>"
  Bus Selector/1 -> Bus Selector1/1  "<chanAndTvalid>"
  CIC Compiler 4.0 3/3 -> Scale/1
  CIC Compiler 4.0 1/3 -> Scale1/1
  CIC Compiler 4.0 2/3 -> Scale2/1
  CIC Compiler 4.0 4/3 -> Scale3/1
  Demux4/1 -> CIC Compiler 4.0 5/2
  Demux4/2 -> CIC Compiler 4.0 6/2
  CIC Compiler 4.0 7/3 -> Scale4/1
  CIC Compiler 4.0 8/3 -> Scale5/1
  CIC Compiler 4.0 9/3 -> Scale6/1
  CIC Compiler 4.0 10/3 -> Scale7/1
  Mux1/1 -> Bus Creator/2  "I&Qlpf"
  Bus Creator/1 -> Out1/1
  Bus Creator1/1 -> Bus Creator/1, Bus Selector2/1  "channel&tvalid"
  CIC Compiler 4.0 7/2 -> Bus Creator1/2  "tvalid"
  CIC Compiler 4.0 7/6 -> Bus Creator1/1  "channel"
  CIC reset/1(notResetOut) -> CIC Compiler 4.0 11/4, CIC Compiler 4.0 12/4, CIC Compiler 4.0 3/4, CIC Compiler 4.0 1/4, CIC Compiler 4.0 2/4, CIC Compiler 4.0 4/4, CIC Compiler 4.0 5/4, CIC Compiler 4.0 6/4, CIC Compiler 4.0 7/4, CIC Compiler 4.0 8/4, CIC Compiler 4.0 9/4, CIC Compiler 4.0 10/4, Gateway Out18/1
  Constant4/1 -> CIC reset/3(N-2)
  [fpgaReset] -> Gateway Out14/1, CIC reset/1(resetIn)
  CIC reset/2(tlast) -> CIC Compiler 4.0 11/3, CIC Compiler 4.0 12/3, CIC Compiler 4.0 3/3, CIC Compiler 4.0 2/3, CIC Compiler 4.0 5/3, CIC Compiler 4.0 6/3, CIC Compiler 4.0 8/3, CIC Compiler 4.0 9/3, CIC Compiler 4.0 10/3, CIC Compiler 4.0 7/3, CIC Compiler 4.0 4/3, CIC Compiler 4.0 1/3, Gateway Out17/1
  Gateway Out18/1 -> CIC LPF input scope/5
  Gateway Out17/1 -> CIC LPF input scope/4
  Gateway Out16/1 -> CIC LPF input scope/3
  Gateway Out15/1 -> CIC LPF input scope/2
  Gateway Out14/1 -> CIC LPF input scope/1
  Bus Selector2/2 -> Gateway Out13/1  "<tvalid>"
  Bus Selector2/1 -> Gateway Out12/1  "<channel>"
  Gateway Out12/1 -> Mux/1
  Gateway Out13/1 -> Mux/2
  Mux/1 -> LPF chan output/1
  Gateway Out/1 -> LPF chan output/2, Display/1
  CIC Compiler 4.0 5/3 -> Scale8/1
  CIC Compiler 4.0 6/3 -> Scale9/1
  Demux2/2 -> CIC Compiler 4.0 11/2
  Demux2/1 -> Gateway Out16/1, CIC Compiler 4.0 12/2
  Scale7/1 -> Mux1/12
  Scale6/1 -> Mux1/11
  Scale5/1 -> Mux1/10
  Scale4/1 -> Mux1/9
  Scale9/1 -> Mux1/8
  Scale8/1 -> Mux1/7
  Scale3/1 -> Mux1/6
  CIC Compiler 4.0 6/6 -> Gateway Out/1
  Scale2/1 -> Mux1/5
  Scale1/1 -> Mux1/4
  Scale/1 -> Mux1/3
  CIC Compiler 4.0 11/3 -> Scale10/1
  CIC Compiler 4.0 12/3 -> Scale11/1
  Scale11/1 -> Mux1/1
  Scale10/1 -> Mux1/2
  CIC Compiler 4.0 1/1 -> Terminator/1
  CIC Compiler 4.0 1/2 -> Terminator1/1
  CIC Compiler 4.0 1/4 -> Terminator2/1
  CIC Compiler 4.0 1/5 -> Terminator3/1
  CIC Compiler 4.0 1/6 -> Terminator4/1
  CIC Compiler 4.0 1/7 -> Terminator5/1
  CIC Compiler 4.0 1/8 -> Terminator6/1
  CIC Compiler 4.0 10/1 -> Terminator7/1
  CIC Compiler 4.0 10/2 -> Terminator8/1
  CIC Compiler 4.0 10/4 -> Terminator9/1
  CIC Compiler 4.0 10/5 -> Terminator10/1
  CIC Compiler 4.0 10/6 -> Terminator11/1
  CIC Compiler 4.0 10/7 -> Terminator12/1
  CIC Compiler 4.0 10/8 -> Terminator13/1
  CIC Compiler 4.0 11/1 -> Terminator14/1
  CIC Compiler 4.0 11/2 -> Terminator15/1
  CIC Compiler 4.0 11/4 -> Terminator16/1
  CIC Compiler 4.0 11/5 -> Terminator17/1
  CIC Compiler 4.0 11/6 -> Terminator18/1
  CIC Compiler 4.0 11/7 -> Terminator19/1
  CIC Compiler 4.0 11/8 -> Terminator20/1
  CIC Compiler 4.0 12/1 -> Terminator21/1
  CIC Compiler 4.0 12/2 -> Terminator22/1
  CIC Compiler 4.0 12/4 -> Terminator23/1
  CIC Compiler 4.0 12/5 -> Terminator24/1
  CIC Compiler 4.0 12/6 -> Terminator25/1
  CIC Compiler 4.0 12/7 -> Terminator26/1
  CIC Compiler 4.0 12/8 -> Terminator27/1
  CIC Compiler 4.0 2/1 -> Terminator28/1
  CIC Compiler 4.0 2/2 -> Terminator29/1
  CIC Compiler 4.0 2/4 -> Terminator30/1
  CIC Compiler 4.0 2/5 -> Terminator31/1
  CIC Compiler 4.0 2/6 -> Terminator32/1
  CIC Compiler 4.0 2/7 -> Terminator33/1
  CIC Compiler 4.0 2/8 -> Terminator34/1
  CIC Compiler 4.0 3/1 -> Terminator35/1
  CIC Compiler 4.0 3/2 -> Terminator36/1
  CIC Compiler 4.0 3/4 -> Terminator37/1
  CIC Compiler 4.0 3/5 -> Terminator38/1
  CIC Compiler 4.0 3/6 -> Terminator39/1
  CIC Compiler 4.0 3/7 -> Terminator40/1
  CIC Compiler 4.0 3/8 -> Terminator41/1
  CIC Compiler 4.0 4/1 -> Terminator42/1
  CIC Compiler 4.0 4/2 -> Terminator43/1
  CIC Compiler 4.0 4/4 -> Terminator44/1
  CIC Compiler 4.0 4/5 -> Terminator45/1
  CIC Compiler 4.0 4/6 -> Terminator46/1
  CIC Compiler 4.0 4/7 -> Terminator47/1
  CIC Compiler 4.0 4/8 -> Terminator48/1
  CIC Compiler 4.0 5/1 -> Terminator49/1
  CIC Compiler 4.0 5/2 -> Terminator50/1
  CIC Compiler 4.0 5/4 -> Terminator51/1
  CIC Compiler 4.0 5/5 -> Terminator52/1
  CIC Compiler 4.0 5/6 -> Terminator53/1
  CIC Compiler 4.0 5/7 -> Terminator54/1
  CIC Compiler 4.0 5/8 -> Terminator55/1
  CIC Compiler 4.0 6/1 -> Terminator56/1
  CIC Compiler 4.0 6/2 -> Terminator57/1
  CIC Compiler 4.0 6/4 -> Terminator58/1
  CIC Compiler 4.0 6/5 -> Terminator59/1
  CIC Compiler 4.0 6/7 -> Terminator60/1
  CIC Compiler 4.0 6/8 -> Terminator61/1
  CIC Compiler 4.0 7/1 -> Terminator62/1
  CIC Compiler 4.0 7/4 -> Terminator63/1
  CIC Compiler 4.0 7/5 -> Terminator64/1
  CIC Compiler 4.0 7/7 -> Terminator65/1
  CIC Compiler 4.0 7/8 -> Terminator66/1
  CIC Compiler 4.0 8/1 -> Terminator67/1
  CIC Compiler 4.0 8/2 -> Terminator68/1
  CIC Compiler 4.0 8/4 -> Terminator69/1
  CIC Compiler 4.0 8/5 -> Terminator70/1
  CIC Compiler 4.0 8/6 -> Terminator71/1
  CIC Compiler 4.0 8/7 -> Terminator72/1
  CIC Compiler 4.0 8/8 -> Terminator73/1
  CIC Compiler 4.0 9/1 -> Terminator74/1
  CIC Compiler 4.0 9/2 -> Terminator75/1
  CIC Compiler 4.0 9/4 -> Terminator76/1
  CIC Compiler 4.0 9/5 -> Terminator77/1
  CIC Compiler 4.0 9/6 -> Terminator78/1
  CIC Compiler 4.0 9/7 -> Terminator79/1
  CIC Compiler 4.0 9/8 -> Terminator80/1

== system CryoDet/DspCore/AdcDac 0/Ref Delay ==
  note: Also delay Sideband Local Oscillator I&Q
  note: Delays DAC output data used as Reference for input signal
      | Delay is to compensate for delay of DAC (big), up/downconverter, cable plant, cryostat etc.
      | This is to prevent too much delay mismatch from winding up phase vs. frequency of S21's of sidebands wrt to central line
  In1 : Inport
  Addressable Shift Register{,1..3} (4 alike) : xbsIndex_r4/Addressable Shift Register  infer_latency=on  depth=2  initVector=[0]  en=off  use_behavioral_HDL=on  Optimization=Resource  dbl_ovrd=off  block_type=addrsr
      settings: infoedit="Delay of configurable length.  Any element in the delay line can be addressed and driven onto the output port.<br><br>Hardware notes: Generates fast, compact FIFO-style shift registers or delay lines using SRL16/SRL32 mode of the slice LUTs"
  Demux : Demux  Outputs=2
  Display : Display
      settings: Decimation=128
  Gateway Out : xbsIndex_r4/Gateway Out  inherit_from_input=off  hdl_port=off  rows=1  columns=1  UseAsDAC=off  DACChannel='1'  interface=None  automatic_assignment=on  address_offset=hex2dec('00')  intf_name=''  intf_description=''  timing_constraint=None  locs_specified=off  LOCs={}  io_standard={}  block_type=gatewayout
  Mux : Mux  Inputs=2
  Out1 : Outport
  tag scope: SBIdel=global, SBQdel=global
  wires:
  Addressable Shift Register/1 -> Mux/1
  Addressable Shift Register1/1 -> Mux/2
  In1/1 -> Demux/1
  Demux/2 -> Addressable Shift Register1/1
  Demux/1 -> Addressable Shift Register/1
  [refDel] -> Addressable Shift Register1/2, Addressable Shift Register/2, Gateway Out/1
  Mux/1 -> Out1/1
  Gateway Out/1 -> Display/1
  [SBI] -> Addressable Shift Register2/1
  [SBQ] -> Addressable Shift Register3/1
  [refDel] -> Addressable Shift Register2/2, Addressable Shift Register3/2
  Addressable Shift Register3/1 -> [SBQdel]
  Addressable Shift Register2/1 -> [SBIdel]
